simulink model "driver_monitor_sim_identification"  (R2025b)
settings: Solver=FixedStepAuto  StartTime=0.0  StopTime=inf  FixedStep=0.05  RelTol=1e-3
libraries: simulink x2, dspnetwork x1
settings Model: Creator=chopd  LastModifiedBy=chopd

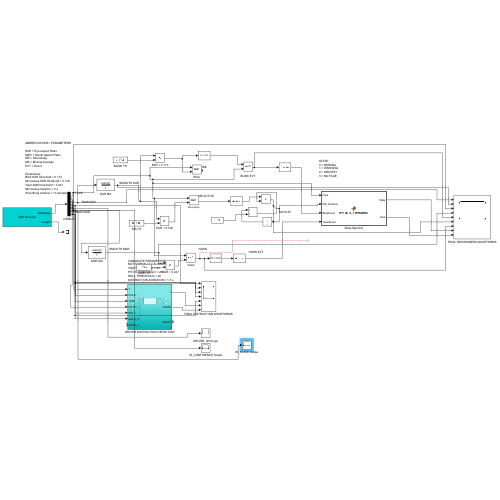
[thumbnail: Simulink's stored preview of the top-level diagram]
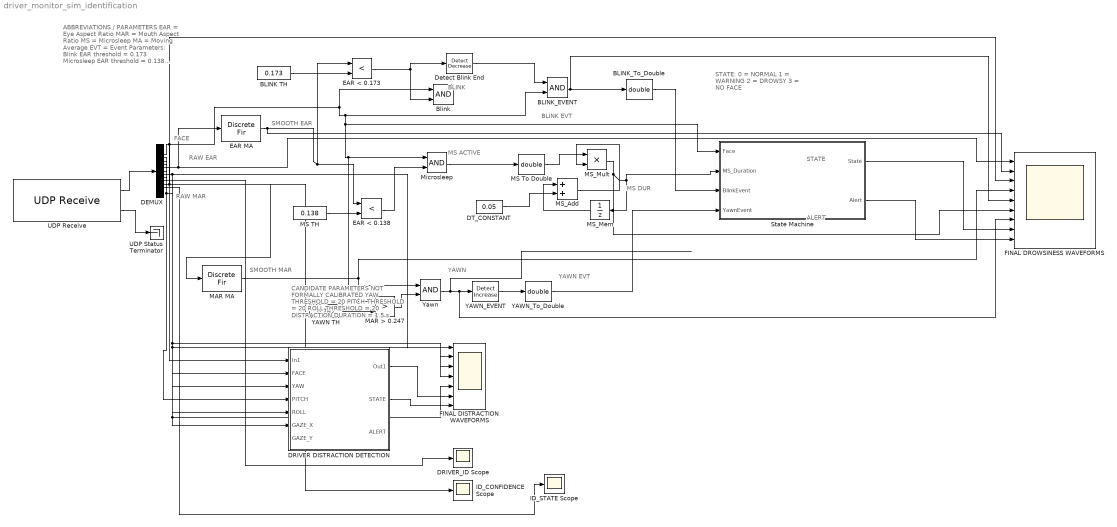
== system driver_monitor_sim_identification ==
  note: ABBREVIATIONS / PARAMETERS
      |
      | EAR = Eye Aspect Ratio
      | MAR = Mouth Aspect Ratio
      | MS = Microsleep
      | MA = Moving Average
      | EVT = Event
      |
      | Parameters:
      | Blink EAR threshold = 0.173
      | Microsleep EAR threshold = 0.138
      | Yawn MAR threshold = 0.247
      | Microsleep duration = 2 s
      | Smoothing window = 10 samples
  note: STATE:
      | 0 = NORMAL
      | 1 = WARNING
      | 2 = DROWSY
      | 3 = NO FACE
  note: FACE
  note: RAW EAR
  note: RAW MAR
  note: SMOOTH EAR
  note: SMOOTH MAR
  note: BLINK
  note: BLINK EVT
  note: MS ACTIVE
  note: MS DUR
  note: YAWN
  note: YAWN EVT
  note: STATE
  note: ALERT
  note: CANDIDATE PARAMETERS
      | NOT FORMALLY CALIBRATED
      | YAW THRESHOLD = 20
      | PITCH THRESHOLD = 20
      | ROLL THRESHOLD = 20
      | DISTRACTION DURATION = 1.5 s
  BLINK TH : Constant  Value=0.173
  BLINK_EVENT : Logic  AllPortsSameDT=off  OutDataTypeStr=boolean
  BLINK_To_Double : DataTypeConversion  OutDataTypeStr=double  SaturateOnIntegerOverflow=off  RndMeth=Floor
  Blink : Logic  AllPortsSameDT=off  OutDataTypeStr=boolean
  DEMUX : Demux  Outputs=11
  DRIVER DISTRACTION DETECTION : Subsystem
  DRIVER_ID Scope : Scope
      settings: ActiveDisplayYMinimum=-1.8312691930845197  ActiveDisplayYMaximum=4.6801569228511326
  DT_CONSTANT : Constant  Value=0.05
  Detect Blink End : simulink/Logic and Bit Operations/Detect Decrease  vinit=0.0  OutDataTypeStr=boolean
  EAR < 0.138 : RelationalOperator  Operator=<  OutDataTypeStr=boolean  RndMeth=Simplest  InputSameDT=off
  EAR < 0.173 : RelationalOperator  Operator=<  OutDataTypeStr=boolean  RndMeth=Simplest  InputSameDT=off
  EAR MA : DiscreteFir  Coefficients=ones(1,10)/10  InitialStates=0.3
  FINAL DISTRACTION WAVEFORMS : Scope  NumInputPorts=7
      settings: Title=YAW|PITCH|ROLL|GAZE_X|GAZE_Y|STATE|ALERT
  FINAL DROWSINESS WAVEFORMS : Scope  NumInputPorts=9
      settings: ActiveDisplayString=9  Title=DROWSINESS ALERT  ActiveDisplayYMinimum=-1  ActiveDisplayYMaximum=1  YLabel=DROWSINESS ALERT
  ID_CONFIDENCE Scope : Scope
      settings: ActiveDisplayYMinimum=0.8536538960674136  ActiveDisplayYMaximum=0.93340500676126226
  ID_STATE Scope : Scope
      settings: ActiveDisplayYMinimum=1  ActiveDisplayYMaximum=3
  MAR > 0.247 : RelationalOperator  Operator=>  OutDataTypeStr=boolean  RndMeth=Simplest  InputSameDT=off
  MAR MA : DiscreteFir  Coefficients=ones(1,10)/10  InitialStates=0.0
  MS TH : Constant  Value=0.138
  MS To Double : DataTypeConversion  OutDataTypeStr=double  SaturateOnIntegerOverflow=off  RndMeth=Floor
  MS_Add : Sum
  MS_Mem : UnitDelay  SampleTime=-1  HasFrameUpgradeWarning=on
  MS_Mult : Product  Inputs=**
  Microsleep : Logic  AllPortsSameDT=off  OutDataTypeStr=boolean
  State Machine : MATLAB Function  TreatAsAtomicUnit=on
  UDP Receive : dspnetwork/UDP Receive  localURL='0.0.0.0'  localPort=5000  remoteURL='0.0.0.0'  remotePort=-1  recvBufferSize=8192  dims=11  signalDatatype=double  isComplex=off  isVarSize=off  showBlockingTime=off  blockingTime=0  sampletime=0.05  blockPlatform=[]
  UDP Status Terminator : Terminator
  YAWN TH : Constant  Value=0.247
  YAWN_EVENT : simulink/Logic and Bit Operations/Detect Increase  vinit=0.0  OutDataTypeStr=boolean
  YAWN_To_Double : DataTypeConversion  OutDataTypeStr=double  SaturateOnIntegerOverflow=off  RndMeth=Floor
  Yawn : Logic  AllPortsSameDT=off  OutDataTypeStr=boolean
  wires:
  UDP Receive/1 -> DEMUX/1
  UDP Receive/2 -> UDP Status Terminator/1
  DEMUX/2 -> EAR MA/1, FINAL DROWSINESS WAVEFORMS/1
  DEMUX/3 -> MAR MA/1, FINAL DROWSINESS WAVEFORMS/3
  MAR MA/1 -> MAR > 0.247/1, FINAL DROWSINESS WAVEFORMS/4
  YAWN TH/1 -> MAR > 0.247/2
  DEMUX/1 -> Yawn/1, Microsleep/1, State Machine/1(Face), BLINK_EVENT/2, Blink/1, DRIVER DISTRACTION DETECTION/1(In1)
  MAR > 0.247/1 -> Yawn/2
  EAR MA/1 -> EAR < 0.138/1, EAR < 0.173/1, FINAL DROWSINESS WAVEFORMS/2
  BLINK TH/1 -> EAR < 0.173/2
  EAR < 0.173/1 -> Blink/2, Detect Blink End/1
  Detect Blink End/1 -> BLINK_EVENT/1
  BLINK_EVENT/1 -> BLINK_To_Double/1, FINAL DROWSINESS WAVEFORMS/5
  BLINK_To_Double/1 -> State Machine/3(BlinkEvent)
  MS TH/1 -> EAR < 0.138/2
  EAR < 0.138/1 -> Microsleep/2
  Microsleep/1 -> MS To Double/1
  MS_Mem/1 -> MS_Add/1
  DT_CONSTANT/1 -> MS_Add/2
  MS_Add/1 -> MS_Mult/2
  MS To Double/1 -> MS_Mult/1
  MS_Mult/1 -> State Machine/2(MS_Duration), MS_Mem/1, FINAL DROWSINESS WAVEFORMS/6
  Yawn/1 -> FINAL DROWSINESS WAVEFORMS/7, YAWN_EVENT/1
  YAWN_EVENT/1 -> YAWN_To_Double/1
  YAWN_To_Double/1 -> State Machine/4(YawnEvent)
  State Machine/1(State) -> FINAL DROWSINESS WAVEFORMS/8
  State Machine/2(Alert) -> FINAL DROWSINESS WAVEFORMS/9
  DEMUX/4 -> DRIVER DISTRACTION DETECTION/2(FACE), FINAL DISTRACTION WAVEFORMS/1
  DEMUX/5 -> DRIVER DISTRACTION DETECTION/3(YAW), FINAL DISTRACTION WAVEFORMS/2
  DEMUX/6 -> DRIVER DISTRACTION DETECTION/4(PITCH), FINAL DISTRACTION WAVEFORMS/3
  DEMUX/7 -> DRIVER DISTRACTION DETECTION/5(ROLL), FINAL DISTRACTION WAVEFORMS/4
  DEMUX/8 -> DRIVER DISTRACTION DETECTION/6(GAZE_X), FINAL DISTRACTION WAVEFORMS/5
  DRIVER DISTRACTION DETECTION/1(Out1) -> FINAL DISTRACTION WAVEFORMS/6
  DRIVER DISTRACTION DETECTION/2(STATE) -> FINAL DISTRACTION WAVEFORMS/7
  DEMUX/9 -> DRIVER_ID Scope/1
  DEMUX/10 -> ID_CONFIDENCE Scope/1
  DEMUX/11 -> ID_STATE Scope/1

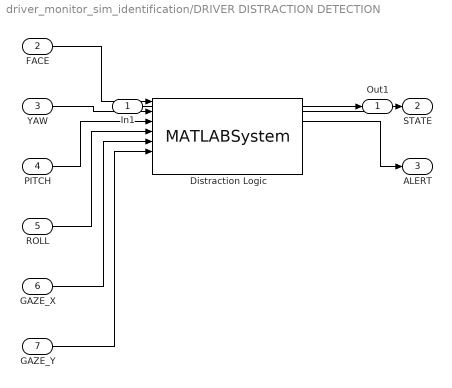
== system driver_monitor_sim_identification/DRIVER DISTRACTION DETECTION ==
  In1 : Inport
  FACE : Inport  Port=2
  YAW : Inport  Port=3
  PITCH : Inport  Port=4
  ROLL : Inport  Port=5
  GAZE_X : Inport  Port=6
  GAZE_Y : Inport  Port=7
  Distraction Logic : MATLABSystem  System=DistractionLogicSystem  YawThreshold=20  PitchThreshold=20  RollThreshold=20  GazeXLeftThreshold=-0.20  GazeXRightThreshold=0.20  GazeYUpThreshold=-0.30  GazeYDownThreshold=0.40  DistractionDuration=1.5  SampleTime=0.05  SimulateUsing=Code generation
      mask Type: DistractionLogicSystem
  Out1 : Outport
  STATE : Outport  Port=2
  ALERT : Outport  Port=3
  wires:
  In1/1 -> Out1/1
  Distraction Logic/1 -> STATE/1
  Distraction Logic/2 -> ALERT/1
  FACE/1 -> Distraction Logic/1
  YAW/1 -> Distraction Logic/2
  PITCH/1 -> Distraction Logic/3
  ROLL/1 -> Distraction Logic/4
  GAZE_X/1 -> Distraction Logic/5
  GAZE_Y/1 -> Distraction Logic/6

== matlab function driver_monitor_sim_identification/State Machine ==
  data: Face input; State output; MS_Duration input; BlinkEvent input; YawnEvent input; Alert output
function [State, Alert] = evaluate_drowsiness(Face, MS_Duration, BlinkEvent, YawnEvent)
    persistent blink_history yawn_history history_idx;
    if isempty(blink_history)
        blink_history = zeros(1200, 1);
        yawn_history = zeros(1200, 1);
        history_idx = 1;
    end
    
    blink_history(history_idx) = BlinkEvent;
    yawn_history(history_idx) = YawnEvent;
    
    history_idx = history_idx + 1;
    if history_idx > 1200
        history_idx = 1;
    end
    
    blink_count = sum(blink_history);
    yawn_count = sum(yawn_history);
    
    MS_THRESH = 2.0;
    BLINK_THRESH = 15;
    YAWN_THRESH = 3;
    
    if Face == 0
        State = 3; % NO_FACE
        Alert = 0;
    elseif MS_Duration >= MS_THRESH
        State = 2; % DROWSY
        Alert = 1;
    elseif yawn_count >= YAWN_THRESH || blink_count >= BLINK_THRESH
        State = 1; % WARNING
        Alert = 0;
    else
        State = 0; % NORMAL
        Alert = 0;
    end
end
